simulink library "cube_lib"  (R2016a)
settings: Solver=VariableStepAuto  StartTime=0.0  StopTime=10.0  RelTol=1e-3
undefined symbols (not defined in the file): noise_standard_deviation, T_test_sensor, test_sensor_seed
libraries: simulink x2
settings Model: Creator=Stefan  LastModifiedBy=Love
settings DataIOCC: LimitDataPoints=on
settings DebuggingCC: AllowSymbolicDim=off
settings ModelReferenceCC: PropagateSignalLabelsOutOfModel=off
settings GRTTargetCC: GeneratePreprocessorConditionals=Use local settings

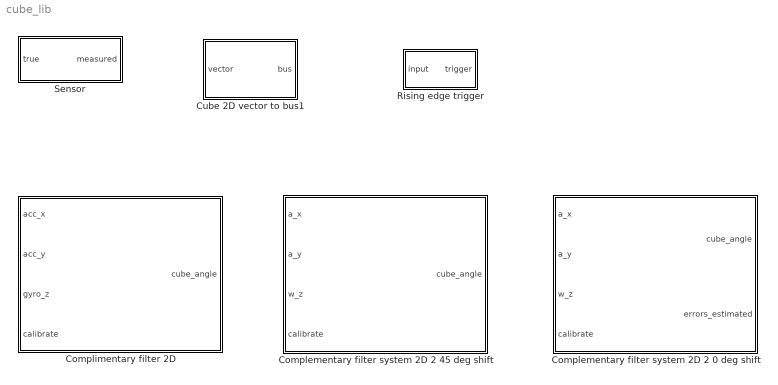
== system cube_lib ==
  Complementary filter system 2D 2 0 deg shift : Subsystem
  Complementary filter system 2D 2 45 deg shift : Subsystem
  Complimentary filter 2D : Subsystem
  Cube 2D vector to bus1 : Subsystem
  Rising edge trigger : Subsystem
  Sensor : Subsystem  mask{scale_factor=1, bias=0, noise_std=noise_standard_deviation, noise_seed=test_sensor_seed, sample_time=T_test_sensor}
      mask prompts: scale_factor "Scale factor"; noise_std "Noise standard deviation"; noise_seed "Noise seed"; sample_time "Sample time"
      mask help:
      | Simulates measurement by adding scale factor error, bias error and noise. Default sensor is a perfect sensor with sampling frequency 10 Hz.
      | Scale factor: 1
      | Bias: 0
      | Noise standard deviation: 0
      |
      | The sensor block contains the "Band-Limited White Noise" block which uses noise power instead of noise standard deviation. Noise power has the following definition:
      | noise_power = T_sample*standard_deviation^2
      | The white noise block has a correlation time of 0, meaning that all values are independent of each other, that is, white noise. (Simulink documentation for this block is confusion on this topic.)
      |
      | Due to the noise generator, sample time cannot be inherited.
      mask Callback sample_time:
      | sample_time_local = str2num(get_param(gcb,'sample_time'));
      | 
      | if sample_time_local <= 0
      |     msgbox(['Invalid setting for sample_time' char(10) ...
      |         'Due to noise generator, sample time cannot be inherited' char(10)...
      |         '(Yes, I know, it''s stupid!)']...
      |         ,'Error','error');
      |     set_param(gcb,'sample_time',num2str(0.1));
      | end

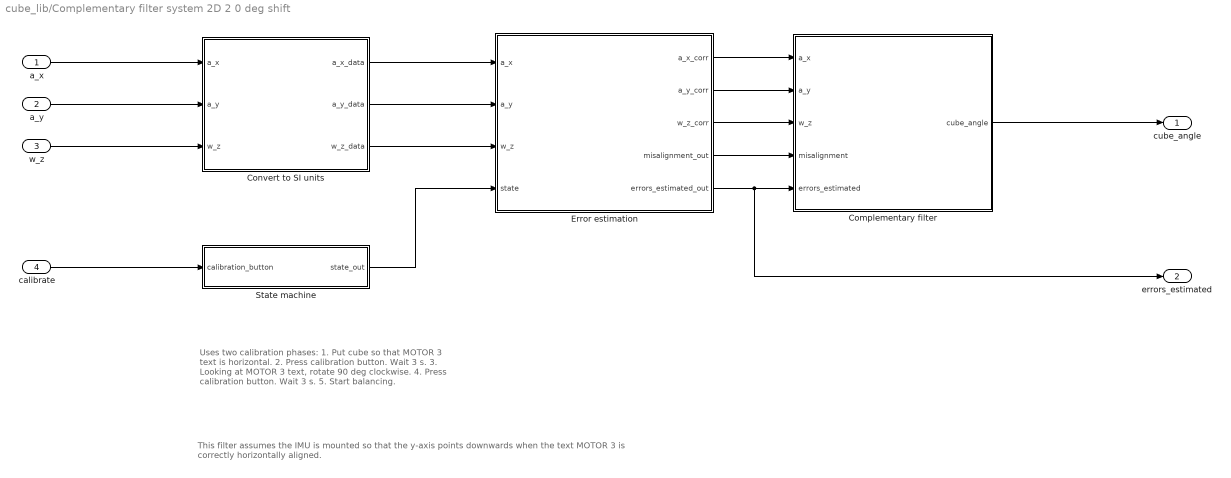
== system cube_lib/Complementary filter system 2D 2 0 deg shift ==
  note: This filter assumes the IMU is mounted so that the y-axis points downwards when the text MOTOR 3 is correctly horizontally aligned.
  note: Uses two calibration phases:
      | 1. Put cube so that MOTOR 3 text is horizontal.
      | 2. Press calibration button. Wait 3 s.
      | 3. Looking at MOTOR 3 text, rotate 90 deg clockwise.
      | 4. Press calibration button. Wait 3 s.
      | 5. Start balancing.
  a_x : Inport
  a_y : Inport  Port=2
  w_z : Inport  Port=3
  calibrate : Inport  Port=4
  Complementary filter : MATLAB Function  TreatAsAtomicUnit=on
  Convert to SI units : MATLAB Function  TreatAsAtomicUnit=on
  Error estimation : MATLAB Function  TreatAsAtomicUnit=on
  State machine : MATLAB Function  TreatAsAtomicUnit=on
  cube_angle : Outport
  errors_estimated : Outport  Port=2
  wires:
  Complementary filter/1(cube_angle) -> cube_angle/1
  w_z/1 -> Convert to SI units/3(w_z)
  a_x/1 -> Convert to SI units/1(a_x)
  a_y/1 -> Convert to SI units/2(a_y)
  Convert to SI units/1(a_x_data) -> Error estimation/1(a_x)
  Convert to SI units/2(a_y_data) -> Error estimation/2(a_y)
  Convert to SI units/3(w_z_data) -> Error estimation/3(w_z)
  Error estimation/1(a_x_corr) -> Complementary filter/1(a_x)
  Error estimation/5(errors_estimated_out) -> Complementary filter/5(errors_estimated), errors_estimated/1
  Error estimation/2(a_y_corr) -> Complementary filter/2(a_y)
  Error estimation/3(w_z_corr) -> Complementary filter/3(w_z)
  Error estimation/4(misalignment_out) -> Complementary filter/4(misalignment)
  calibrate/1 -> State machine/1(calibration_button)
  State machine/1(state_out) -> Error estimation/4(state)

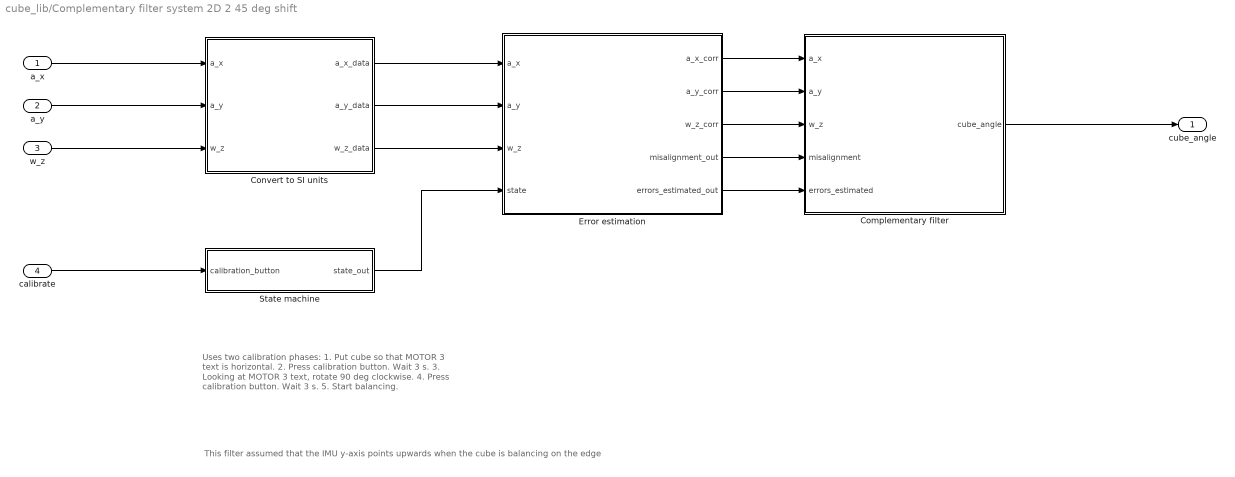
== system cube_lib/Complementary filter system 2D 2 45 deg shift ==
  note: This filter assumed that the IMU y-axis points upwards when the cube is balancing on the edge
  note: Uses two calibration phases:
      | 1. Put cube so that MOTOR 3 text is horizontal.
      | 2. Press calibration button. Wait 3 s.
      | 3. Looking at MOTOR 3 text, rotate 90 deg clockwise.
      | 4. Press calibration button. Wait 3 s.
      | 5. Start balancing.
  a_x : Inport
  a_y : Inport  Port=2
  w_z : Inport  Port=3
  calibrate : Inport  Port=4
  Complementary filter : MATLAB Function  TreatAsAtomicUnit=on
  Convert to SI units : MATLAB Function  TreatAsAtomicUnit=on
  Error estimation : MATLAB Function  TreatAsAtomicUnit=on
  State machine : MATLAB Function  TreatAsAtomicUnit=on
  cube_angle : Outport
  wires:
  State machine/1(state_out) -> Error estimation/4(state)
  calibrate/1 -> State machine/1(calibration_button)
  Error estimation/4(misalignment_out) -> Complementary filter/4(misalignment)
  Error estimation/3(w_z_corr) -> Complementary filter/3(w_z)
  Error estimation/2(a_y_corr) -> Complementary filter/2(a_y)
  Complementary filter/1(cube_angle) -> cube_angle/1
  Error estimation/5(errors_estimated_out) -> Complementary filter/5(errors_estimated)
  Error estimation/1(a_x_corr) -> Complementary filter/1(a_x)
  Convert to SI units/3(w_z_data) -> Error estimation/3(w_z)
  Convert to SI units/2(a_y_data) -> Error estimation/2(a_y)
  Convert to SI units/1(a_x_data) -> Error estimation/1(a_x)
  a_y/1 -> Convert to SI units/2(a_y)
  a_x/1 -> Convert to SI units/1(a_x)
  w_z/1 -> Convert to SI units/3(w_z)

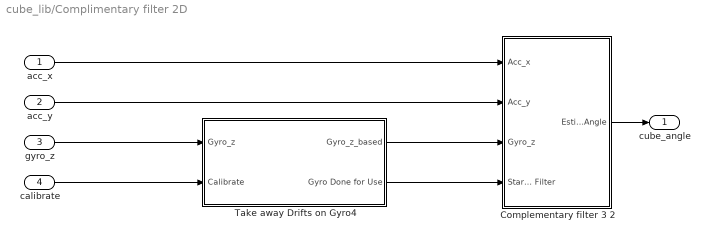
== system cube_lib/Complimentary filter 2D ==
  acc_x : Inport
  acc_y : Inport  Port=2
  gyro_z : Inport  Port=3
  calibrate : Inport  Port=4
  Complementary filter 3 2 : Subsystem
  Take away Drifts on Gyro4 : Subsystem
  cube_angle : Outport
  wires:
  calibrate/1 -> Take away Drifts on Gyro4/2(Calibrate)
  acc_y/1 -> Complementary filter 3 2/2(Acc_y)
  gyro_z/1 -> Take away Drifts on Gyro4/1(Gyro_z)
  acc_x/1 -> Complementary filter 3 2/1(Acc_x)
  Take away Drifts on Gyro4/2(Gyro Done for Use) -> Complementary filter 3 2/4("Start Complementary Filter ")
  Complementary filter 3 2/1(Estimated_Angle) -> cube_angle/1
  Take away Drifts on Gyro4/1(Gyro_z_based) -> Complementary filter 3 2/3(Gyro_z)

== system cube_lib/Cube 2D vector to bus1 ==
  vector : Inport
  Bus Creator1 : BusCreator  Inputs=5  OutDataTypeStr=Bus: CubeStates2D
  Demux2 : Demux  Outputs=5
  bus : Outport
  wires:
  vector/1 -> Demux2/1
  Demux2/3 -> Bus Creator1/3  "cube_angular_acceleration"
  Demux2/4 -> Bus Creator1/4  "wheel_angular_velocity"
  Demux2/5 -> Bus Creator1/5  "wheel_angular_acceleration"
  Demux2/2 -> Bus Creator1/2  "cube_angular_velocity"
  Demux2/1 -> Bus Creator1/1  "cube_angle"
  Bus Creator1/1 -> bus/1

== system cube_lib/Rising edge trigger ==
  input : Inport
  Compare To Zero : simulink/Logic and Bit Operations/Compare To Zero  relop=>  OutDataTypeStr=boolean
  Delay3 : Delay  DelayLength=1  InitialCondition=0
  Sum : Sum  Inputs=+-
  trigger : Outport
  wires:
  input/1 -> Sum/1, Delay3/1
  Delay3/1 -> Sum/2
  Compare To Zero/1 -> trigger/1
  Sum/1 -> Compare To Zero/1

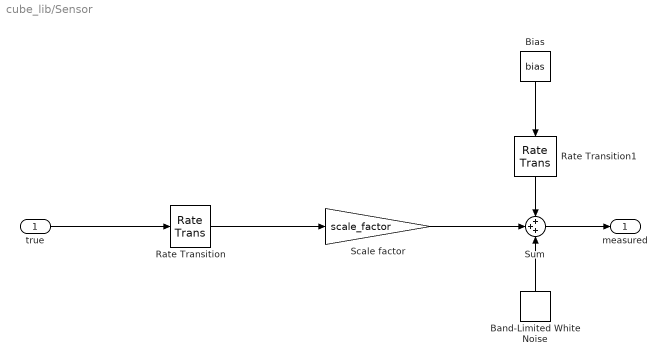
== system cube_lib/Sensor ==
  true : Inport
  Band-Limited White Noise : simulink/Sources/Band-Limited White Noise  Cov=sample_time*noise_std^2  Ts=sample_time  seed=noise_seed
  Bias : Constant  Value=bias
  Rate Transition : RateTransition  OutPortSampleTime=sample_time
  Rate Transition1 : RateTransition  OutPortSampleTime=sample_time
  Scale factor : Gain  Gain=scale_factor
  Sum : Sum  Inputs=+++
  measured : Outport
  wires:
  Rate Transition/1 -> Scale factor/1
  true/1 -> Rate Transition/1
  Sum/1 -> measured/1
  Scale factor/1 -> Sum/2
  Band-Limited White Noise/1 -> Sum/3
  Bias/1 -> Rate Transition1/1
  Rate Transition1/1 -> Sum/1

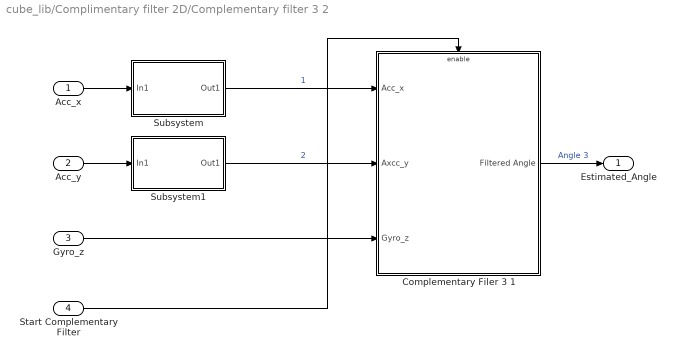
== system cube_lib/Complimentary filter 2D/Complementary filter 3 2 ==
  Acc_x : Inport
  Acc_y : Inport  Port=2
  Gyro_z : Inport  Port=3
  "Start Complementary Filter " : Inport  Port=4
  Complementary Filer 3 1 : Subsystem
  Subsystem : Subsystem
  Subsystem1 : Subsystem
  Estimated_Angle : Outport
  wires:
  Acc_x/1 -> Subsystem/1(In1)
  Acc_y/1 -> Subsystem1/1(In1)
  Complementary Filer 3 1/1(Filtered Angle) -> Estimated_Angle/1  "Angle 3"
  "Start Complementary Filter "/1 -> Complementary Filer 3 1/Enable
  Gyro_z/1 -> Complementary Filer 3 1/3(Gyro_z)
  Subsystem1/1(Out1) -> Complementary Filer 3 1/2(Axcc_y)  "2"
  Subsystem/1(Out1) -> Complementary Filer 3 1/1(Acc_x)  "1"

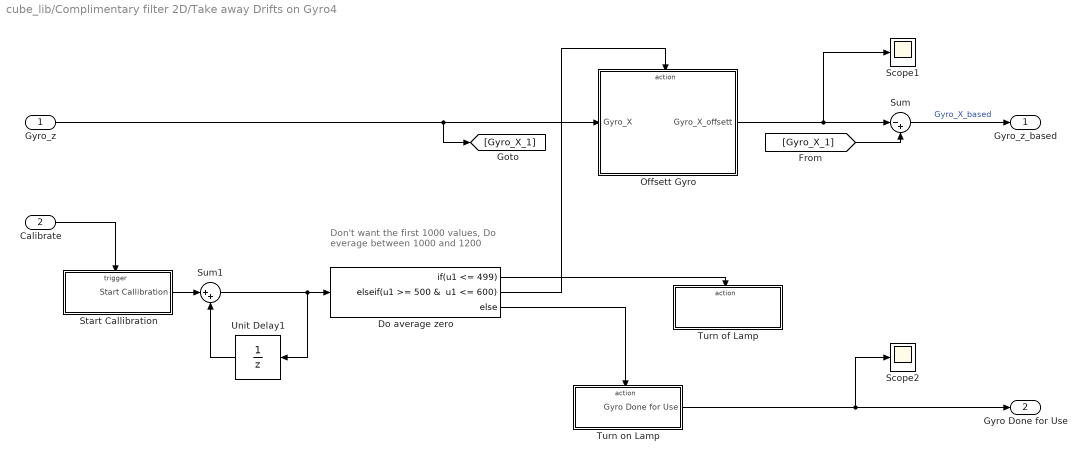
== system cube_lib/Complimentary filter 2D/Take away Drifts on Gyro4 ==
  note: Don't want the first 1000 values,
      | Do everage between 1000 and 1200
  Gyro_z : Inport
  Calibrate : Inport  Port=2
  Do average zero : If  IfExpression=u1 <= 499  ElseIfExpressions="u1 >= 500 &  u1 <= 600"
  Offsett Gyro : Subsystem
  Scope1 : Scope
  Scope2 : Scope
  Start Callibration : Subsystem
  Sum : Sum  Inputs=|-+
  Sum1 : Sum  Inputs=|++
  Turn of Lamp : Subsystem
  Turn on Lamp : Subsystem
  Unit Delay1 : UnitDelay  SampleTime=-1
  Gyro_z_based : Outport
  Gyro Done for Use : Outport  Port=2
  wires:
  Turn on Lamp/1(Gyro Done for Use) -> Gyro Done for Use/1, Scope2/1
  Do average zero/1 -> Turn of Lamp/Action
  Start Callibration/1(Start Callibration) -> Sum1/1
  Calibrate/1 -> Start Callibration/Trigger
  Do average zero/3 -> Turn on Lamp/Action
  Do average zero/2 -> Offsett Gyro/Action
  Gyro_z/1 -> Offsett Gyro/1(Gyro_X), [Gyro_X_1]
  Sum/1 -> Gyro_z_based/1  "Gyro_X_based"
  Offsett Gyro/1(Gyro_X_offsett) -> Sum/1, Scope1/1
  [Gyro_X_1] -> Sum/2
  Sum1/1 -> Unit Delay1/1, Do average zero/1
  Unit Delay1/1 -> Sum1/2

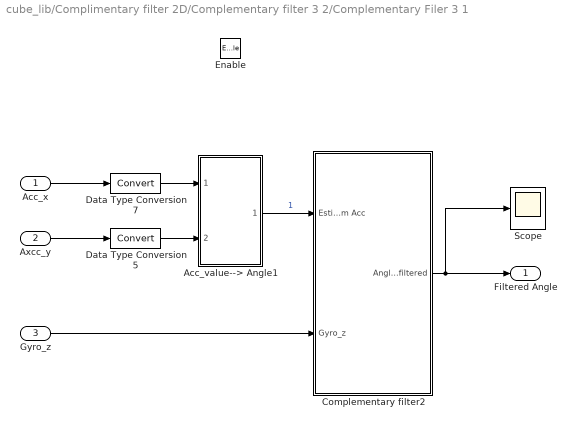
== system cube_lib/Complimentary filter 2D/Complementary filter 3 2/Complementary Filer 3 1 ==
  Acc_x : Inport
  Axcc_y : Inport  Port=2
  Gyro_z : Inport  Port=3
  Enable : EnablePort  StatesWhenEnabling=reset
  Acc_value--> Angle1 : Subsystem
  Complementary filter2 : Subsystem
  Data Type Conversion5 : DataTypeConversion
  Data Type Conversion7 : DataTypeConversion
  Scope : Scope
  Filtered Angle : Outport  OutputWhenDisabled=reset  InitialOutput=[0]
  wires:
  Gyro_z/1 -> Complementary filter2/2(Gyro_z)
  Data Type Conversion5/1 -> Acc_value--> Angle1/2(Acc_y)
  Data Type Conversion7/1 -> Acc_value--> Angle1/1(Acc_x)
  Axcc_y/1 -> Data Type Conversion5/1
  Acc_value--> Angle1/1(Angle) -> Complementary filter2/1(Estimated angle from Acc)  "1"
  Acc_x/1 -> Data Type Conversion7/1
  Complementary filter2/1(Angle_filtered) -> Filtered Angle/1, Scope/1

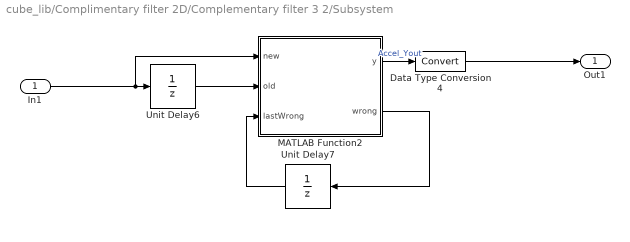
== system cube_lib/Complimentary filter 2D/Complementary filter 3 2/Subsystem ==
  In1 : Inport
  Data Type Conversion4 : DataTypeConversion
  MATLAB Function2 : MATLAB Function  TreatAsAtomicUnit=on
  Unit Delay6 : UnitDelay  InitialCondition=-40.45  SampleTime=-1
  Unit Delay7 : UnitDelay  SampleTime=-1
  Out1 : Outport
  wires:
  In1/1 -> Unit Delay6/1, MATLAB Function2/1(new)
  MATLAB Function2/1(y) -> Data Type Conversion4/1  "Accel_Yout"
  MATLAB Function2/2(wrong) -> Unit Delay7/1
  Unit Delay6/1 -> MATLAB Function2/2(old)
  Unit Delay7/1 -> MATLAB Function2/3(lastWrong)
  Data Type Conversion4/1 -> Out1/1

== system cube_lib/Complimentary filter 2D/Complementary filter 3 2/Subsystem1 ==
  In1 : Inport
  Data Type Conversion4 : DataTypeConversion
  MATLAB Function2 : MATLAB Function  TreatAsAtomicUnit=on
  Unit Delay6 : UnitDelay  InitialCondition=-40.45  SampleTime=-1
  Unit Delay7 : UnitDelay  SampleTime=-1
  Out1 : Outport
  wires:
  In1/1 -> Unit Delay6/1, MATLAB Function2/1(new)
  MATLAB Function2/1(y) -> Data Type Conversion4/1  "Accel_Yout"
  MATLAB Function2/2(wrong) -> Unit Delay7/1
  Unit Delay6/1 -> MATLAB Function2/2(old)
  Unit Delay7/1 -> MATLAB Function2/3(lastWrong)
  Data Type Conversion4/1 -> Out1/1

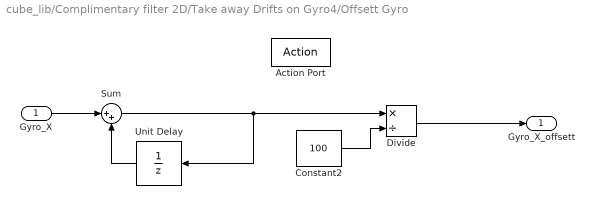
== system cube_lib/Complimentary filter 2D/Take away Drifts on Gyro4/Offsett Gyro ==
  Gyro_X : Inport
  Action Port : ActionPort
  Constant2 : Constant  Value=100
  Divide : Product  Inputs=*/
  Sum : Sum  Inputs=|++
  Unit Delay : UnitDelay  SampleTime=-1
  Gyro_X_offsett : Outport
  wires:
  Sum/1 -> Unit Delay/1, Divide/1
  Divide/1 -> Gyro_X_offsett/1
  Gyro_X/1 -> Sum/1
  Constant2/1 -> Divide/2
  Unit Delay/1 -> Sum/2

== system cube_lib/Complimentary filter 2D/Take away Drifts on Gyro4/Start Callibration ==
  Trigger : TriggerPort  VariantControl=Variant  PortDimensions=1
  Constant2 : Constant
  Start Callibration : Outport  InitialOutput=[0]
  wires:
  Constant2/1 -> Start Callibration/1

== system cube_lib/Complimentary filter 2D/Take away Drifts on Gyro4/Turn of Lamp ==
  Action Port : ActionPort

== system cube_lib/Complimentary filter 2D/Take away Drifts on Gyro4/Turn on Lamp ==
  Action Port : ActionPort
  Constant6 : Constant  SampleTime=-1
  Gyro Done for Use : Outport  InitialOutput=[0]
  wires:
  Constant6/1 -> Gyro Done for Use/1

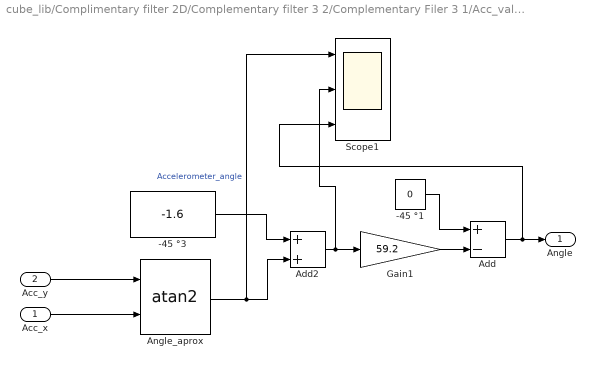
== system cube_lib/Complimentary filter 2D/Complementary filter 3 2/Complementary Filer 3 1/Acc_value--> Angle1 ==
  Acc_x : Inport
  Acc_y : Inport  Port=2
  -45 °1 : Constant  Value=0
  -45 °3 : Constant  Value=-1.6
  Add : Sum  Inputs=+-
  Add2 : Sum
  Angle_aprox : Trigonometry  Operator=atan2
  Gain1 : Gain  Gain=59.2
  Scope1 : Scope  NumInputPorts=3
  Angle : Outport
  wires:
  Add2/1 -> Gain1/1, Scope1/2
  Angle_aprox/1 -> Add2/2, Scope1/1  "Accelerometer_angle"
  -45 °3/1 -> Add2/1
  -45 °1/1 -> Add/1
  Add/1 -> Angle/1, Scope1/3
  Gain1/1 -> Add/2
  Acc_x/1 -> Angle_aprox/2
  Acc_y/1 -> Angle_aprox/1

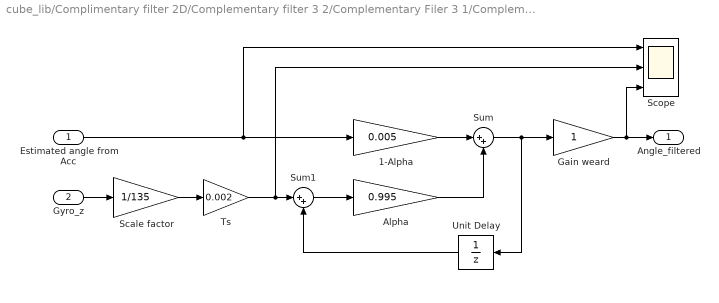
== system cube_lib/Complimentary filter 2D/Complementary filter 3 2/Complementary Filer 3 1/Complementary filter2 ==
  Estimated angle from Acc : Inport
  Gyro_z : Inport  Port=2
  1-Alpha : Gain  Gain=0.005
  Alpha : Gain  Gain=0.995
  Gain weard : Gain
  Scale factor : Gain  Gain=1/135
  Scope : Scope  NumInputPorts=3
  Sum : Sum  Inputs=|++
  Sum1 : Sum  Inputs=|++
  Ts : Gain  Gain=0.002
  Unit Delay : UnitDelay  SampleTime=-1
  Angle_filtered : Outport
  wires:
  Scale factor/1 -> Ts/1
  Sum/1 -> Unit Delay/1, Gain weard/1
  Gain weard/1 -> Scope/3, Angle_filtered/1
  Estimated angle from Acc/1 -> 1-Alpha/1, Scope/1
  Gyro_z/1 -> Scale factor/1
  Unit Delay/1 -> Sum1/2
  Alpha/1 -> Sum/2
  Sum1/1 -> Alpha/1
  Ts/1 -> Sum1/1, Scope/2
  1-Alpha/1 -> Sum/1

== matlab function cube_lib/Complementary filter system 2D 2 0 deg shift/Complementary filter ==
  data: a_x input size=1; a_y input size=1; w_z input size=1; misalignment input size=1; cube_angle output; errors_estimated input size=1
function cube_angle = ComplementaryFilter(a_x,a_y,w_z,misalignment,errors_estimated)
%#codegen
% Uses the equation:
% theta(k) = alfa*(theta(k-1) + w_z*T) + (1-alfa)*a(k);
% where a(k) is the estimated angle from the accelerometers
%
% alfa from cubeparameters

persistent theta_k_1; % Previous cube angle
persistent initiate_filter;

alfa = 0.995;
T_onboard = 0.002;
angle_correction = 135*pi/180; % Due to mounting

if isempty(theta_k_1)
    initiate_filter = 1;
    theta_k_1 = 0;
end

if errors_estimated && initiate_filter % First call to complementary filter (when no previous value exists)
    theta = atan2(a_x,a_y)-misalignment;
    initiate_filter = 0;
elseif errors_estimated
    % Complementary filter
    a_k = atan2(a_x,a_y)-misalignment; % Angle estimation from accelerometers
    % Improvement: Compensate for angular acceleration and centripetal
    % force
    theta = alfa*(theta_k_1 + w_z*T_onboard) + (1-alfa)*a_k;
else
    theta = 0;
end

theta_k_1 = theta;  % Save value

% Assign output
if errors_estimated
    cube_angle = theta + angle_correction;
else
    cube_angle = 0;
end

== matlab function cube_lib/Complementary filter system 2D 2 0 deg shift/Convert to SI units ==
  data: a_x input; a_x_data output double; a_y input; w_z input; a_y_data output double; w_z_data output double
function [a_x_data,a_y_data,w_z_data] = ConvertImuData(a_x,a_y,w_z)
%#codegen

g_ = 9.81*m_/s_^2;
a_scale_factor = 16384; % AFS_SEL = 0, se datablad MPU9250
w_scale_factor = 131;   % FS_SEL = 0, se datablad MPU9250
a_x_data = double(a_x)/a_scale_factor*g_;
a_y_data = double(a_y)/a_scale_factor*g_;
w_z_data = double(w_z)/w_scale_factor*deg_;

== matlab function cube_lib/Complementary filter system 2D 2 0 deg shift/Error estimation ==
  data: a_x input; a_x_corr output; a_y_corr output; w_z_corr output; misalignment_out output; a_y input; w_z input; state input; errors_estimated_out output
function [a_x_corr,a_y_corr,w_z_corr,misalignment_out,errors_estimated_out] = ErrorEstimatedImu(a_x,a_y,w_z,state)
%#codegen
% Finds IMU errors and corrects IMU data
persistent a_x_1; % Vector
persistent a_x_2; % Vector
persistent a_y_1; % Vector
persistent a_y_2; % Vector
persistent w_z_1; % Vector
persistent w_z_2; % Vector
persistent w_z_turn; % Scalar (sum)
persistent n_samples_w_z_turn; % Counts number of samples used for turn to compensate for bias
persistent k_sample;
persistent previous_state;
persistent errors_estimated;
persistent bias_a_x;
persistent bias_a_y;
persistent bias_w_z;
persistent scale_factor_a_x;
persistent scale_factor_a_y;
persistent scale_factor_w_z;
persistent misalignment;

n_samples = 1000; % Two seconds with T=0.002. Hardcoded for compiler
T_onboard = 0.002; % So that it does not have to be input or a set parameter

if isempty(a_x_1)
    k_sample = 1;
    previous_state = 0;
    errors_estimated = 0;
    a_x_1 = zeros(n_samples,1);
    a_x_2 = zeros(n_samples,1);
    a_y_1 = zeros(n_samples,1);
    a_y_2 = zeros(n_samples,1);
    w_z_1 = zeros(n_samples,1);
    w_z_2 = zeros(n_samples,1);
    w_z_turn = 0;
    n_samples_w_z_turn = 0;
    bias_a_x = 0;
    bias_a_y = 0;
    bias_w_z = 0;
    scale_factor_a_x = 0;
    scale_factor_a_y = 0;
    scale_factor_w_z = 0;
    misalignment = 0;
end

if state ~= previous_state % Entering a new state
    k_sample = 1;
    if state == 0 % Start over
        errors_estimated = 0;
        a_x_1 = zeros(n_samples,1);
        a_x_2 = zeros(n_samples,1);
        a_y_1 = zeros(n_samples,1);
        a_y_2 = zeros(n_samples,1);
        w_z_1 = zeros(n_samples,1);
        w_z_2 = zeros(n_samples,1);
        w_z_turn = 0;
        n_samples_w_z_turn = 0;
        bias_a_x = 0;
        bias_a_y = 0;
        bias_w_z = 0;
        scale_factor_a_x = 0;
        scale_factor_a_y = 0;
        scale_factor_w_z = 0;
        misalignment = 0;
    end
end

% Collect data in two phases, where cube_angle = -45 deg and cube_angle = 45 deg
if state == 1 && k_sample <= n_samples
    a_x_1(k_sample) = a_x;
    a_y_1(k_sample) = a_y;
    w_z_1(k_sample) = w_z;
    k_sample = k_sample + 1;
elseif state == 1
    w_z_turn = w_z_turn + w_z;
    n_samples_w_z_turn = n_samples_w_z_turn + 1;
    
end

if state == 2 && k_sample <= n_samples
    a_x_2(k_sample) = a_x;
    a_y_2(k_sample) = a_y;
    w_z_2(k_sample) = w_z;
    k_sample = k_sample + 1;
end

% Estimate errors when data from the two fixed positions have been done
if state == 2 && k_sample > n_samples && ~errors_estimated % We can estimate the errors
    % Sections
    a_x_1_meas = mean(a_x_1);
    a_x_2_meas = mean(a_x_2);
    a_y_1_meas = mean(a_y_1);
    a_y_2_meas = mean(a_y_2);
    w_z_meas   = mean([w_z_1;w_z_2]);
    
    % Call error estimation function
    % Derive expressions from this equations system:
    %  / a_1_measured = scale_factor*a_2_true + bias
    % {
    %  \ a_2_measured = scale_factor*a_2_true + bias
    g = 9.81;
    
    % IMU aligned with cube side, so that the y-axis points downwards when
    % the text MOTOR 3 is correctly horizontally aligned
    % First position:  a_x = 0, a_y = g
    % Second position: a_x = g, a_y = 0
    % That means:
    % a_x_1_meas = bias_x
    % a_x_2_meas = scale_factor_x*-g+bias_x = scale_factor_x*-g + a_x_1_meas
    %   and
    % a_y_1_meas = scale_factor_y*-g+bias_y = scale_factor_y*-g + a_y_1_meas
    % a_y_2_meas = bias_y
    % Great!
    bias_a_x = a_x_1_meas;
    bias_a_y = a_y_2_meas;
    scale_factor_a_x = (a_x_1_meas-a_x_2_meas)/g;
    scale_factor_a_y = (a_y_2_meas-a_y_1_meas)/g;
    
    % Gyro
    bias_w_z = w_z_meas; % Cube is still. What is measured is bias (and error)
    scale_factor_w_z = w_z_turn*T_onboard/(pi/2)-n_samples_w_z_turn*bias_w_z*T_onboard/(pi/2); % Should be a pi/2 turn. Compensate for bias.
    
    % Misalignment
    misalignment = 0;
    
    errors_estimated = 1;
end

% Update
previous_state = state;

% Assign output
if errors_estimated
    a_x_corr = (a_x-bias_a_x)/scale_factor_a_x;
    a_y_corr = (a_y-bias_a_y)/scale_factor_a_y;
    w_z_corr = (w_z-bias_w_z)/scale_factor_w_z;
else
    a_x_corr = a_x;
    a_y_corr = a_y;
    w_z_corr = w_z;
end

misalignment_out = misalignment;
errors_estimated_out = errors_estimated;

== matlab function cube_lib/Complementary filter system 2D 2 0 deg shift/State machine ==
  data: calibration_button input; state_out output
function state_out = StateMachine(calibration_button)
%#codegen
% Step between states 0, 1 and 2 from calibration button

persistent previous_value;
persistent sample;
persistent state;
persistent button_released;

min_samples_between_state_shift = 500; % 500 = 1 s

if isempty(previous_value)
    previous_value = false;
    state = 0;
    sample = min_samples_between_state_shift; % So that button can be clicked instantly
    button_released = true; % Button should be released inbetween clicks
end

if previous_value == 0 && calibration_button == 1 && sample > min_samples_between_state_shift && button_released
    state = state + 1;
    sample = 0;
    button_released = false;
end

if state == 3 % Start over
    state = 0;
end

if previous_value == 1 && calibration_button == 0
    button_released = true;
end

% Increment
sample = sample + 1;
previous_value = calibration_button;

% Assign output
state_out = state;

== matlab function cube_lib/Complementary filter system 2D 2 45 deg shift/Complementary filter ==
  data: a_x input size=1; a_y input size=1; w_z input size=1; misalignment input size=1; cube_angle output; errors_estimated input size=1
function cube_angle = ComplementaryFilter(a_x,a_y,w_z,misalignment,errors_estimated)
%#codegen
% Uses the equation:
% theta(k) = alfa*(theta(k-1) + w_z*T) + (1-alfa)*a(k);
% where a(k) is the estimated angle from the accelerometers
%
% alfa from cubeparameters

persistent theta_k_1; % Previous cube angle
persistent initiate_filter;

alfa = 0.995;
T_onboard = 0.002;

if isempty(theta_k_1)
    initiate_filter = 1;
    theta_k_1 = 0;
end

if errors_estimated && initiate_filter % First call to complementary filter (when no previous value exists)
    theta = atan2(a_x,a_y)-misalignment;
    initiate_filter = 0;
elseif errors_estimated
    % Complementary filter
    a_k = atan2(a_x,a_y)-misalignment; % Angle estimation from accelerometers
    % Improvement: Compensate for angular acceleration and centripetal
    % force
    theta = alfa*(theta_k_1 + w_z*T_onboard) + (1-alfa)*a_k;
else
    theta = 0;
end

theta_k_1 = theta;  % Save value

% Assign output
cube_angle = theta;

== matlab function cube_lib/Complementary filter system 2D 2 45 deg shift/Convert to SI units ==
  data: a_x input; a_x_data output double; a_y input; w_z input; a_y_data output double; w_z_data output double
function [a_x_data,a_y_data,w_z_data] = ConvertImuData(a_x,a_y,w_z)
%#codegen

g_ = 9.81*m_/s_^2;
a_scale_factor = 16384; % AFS_SEL = 0, se datablad MPU9250
w_scale_factor = 131;   % FS_SEL = 0, se datablad MPU9250
a_x_data = double(a_x)/a_scale_factor*g_;
a_y_data = double(a_y)/a_scale_factor*g_;
w_z_data = double(w_z)/w_scale_factor*deg_;

== matlab function cube_lib/Complementary filter system 2D 2 45 deg shift/Error estimation ==
  data: a_x input; a_x_corr output; a_y_corr output; w_z_corr output; misalignment_out output; a_y input; w_z input; state input; errors_estimated_out output
function [a_x_corr,a_y_corr,w_z_corr,misalignment_out,errors_estimated_out] = ErrorEstimatedImu(a_x,a_y,w_z,state)
%#codegen
% Finds IMU errors and corrects IMU data
persistent a_x_1;
persistent a_x_2;
persistent a_y_1;
persistent a_y_2;
persistent w_z_1;
persistent w_z_2;
persistent k_sample;
persistent previous_state;
persistent errors_estimated;
persistent bias_a_x;
persistent bias_a_y;
persistent bias_w_z;
persistent scale_factor_a_x;
persistent scale_factor_a_y;
persistent scale_factor_w_z;
persistent misalignment;

n_samples = 1000; % Two seconds with T=0.002. Hardcoded for compiler

if isempty(a_x_1)
    k_sample = 1;
    previous_state = 0;
    errors_estimated = 0;
    a_x_1 = zeros(n_samples,1);
    a_x_2 = zeros(n_samples,1);
    a_y_1 = zeros(n_samples,1);
    a_y_2 = zeros(n_samples,1);
    w_z_1 = zeros(n_samples,1);
    w_z_2 = zeros(n_samples,1);
    bias_a_x = 0;
    bias_a_y = 0;
    bias_w_z = 0;
    scale_factor_a_x = 0;
    scale_factor_a_y = 0;
    scale_factor_w_z = 0;
    misalignment = 0;
end

if state ~= previous_state % Entering a new state
    k_sample = 1;
end

% Collect data in two sections, where cube_angle = 45 deg and cube_angle = -45 deg
if state == 1 && k_sample <= n_samples
    a_x_1(k_sample) = a_x;
    a_y_1(k_sample) = a_y;
    w_z_1(k_sample) = w_z;
    k_sample = k_sample + 1;
end

if state == 2 && k_sample <= n_samples
    a_x_2(k_sample) = a_x;
    a_y_2(k_sample) = a_y;
    w_z_2(k_sample) = w_z;
    k_sample = k_sample + 1;
end

% Estimate errors when data from the two fixed positions have been done
if state == 2 && k_sample > n_samples && ~errors_estimated % We can estimate the errors
    % Sections
    a_x_1_meas = mean(a_x_1);
    a_x_2_meas = mean(a_x_2);
    a_y_1_meas = mean(a_y_1);
    a_y_2_meas = mean(a_y_2);
    w_z_meas   = mean([w_z_1;w_z_2]);
    
    % Call error estimation function
    [misalignment,...
     bias_a_x,...
     bias_a_y,...
     bias_w_z,...
     scale_factor_a_x,...
     scale_factor_a_y,...
     scale_factor_w_z] = CalculateImuErrors2D(a_x_1_meas,...
                                              a_x_2_meas,...
                                              a_y_1_meas,...
                                              a_y_2_meas,...
                                              w_z_meas);

    errors_estimated = 1;
end

% Update
previous_state = state;

% Assign output
if errors_estimated
    a_x_corr = (a_x-bias_a_x)/scale_factor_a_x;
    a_y_corr = (a_y-bias_a_y)/scale_factor_a_y;
    w_z_corr = (w_z-bias_w_z)/scale_factor_w_z;
else
    a_x_corr = a_x;
    a_y_corr = a_y;
    w_z_corr = w_z;
end

misalignment_out = misalignment;
errors_estimated_out = errors_estimated;

== matlab function cube_lib/Complementary filter system 2D 2 45 deg shift/State machine ==
  data: calibration_button input; state_out output
function state_out = StateMachine(calibration_button)
%#codegen

persistent previous_value;
persistent sample;
persistent state;
persistent button_released;

min_samples_between_state_shift = 500; % 500 = 1 s

if isempty(previous_value)
    previous_value = false;
    state = 0;
    sample = min_samples_between_state_shift; % So that button can be clicked instantly
    button_released = true; % Button should be released inbetween clicks
end

if previous_value == 0 && calibration_button == 1 && sample > min_samples_between_state_shift && button_released
    state = state + 1;
    sample = 0;
    button_released = false;
end

if previous_value == 1 && calibration_button == 0
    button_released = true;
end

% Increment
sample = sample + 1;
previous_value = calibration_button;

% Assign output
state_out = state;

== matlab function cube_lib/Complimentary filter 2D/Complementary filter 3 2/Subsystem/MATLAB Function2 ==
  data: y output; new input; old input; wrong output; lastWrong input
function [y, wrong]= fcn(new, old, lastWrong)
%#codegen
if(old-new > 4000 || new-old > 4000)
    if(lastWrong == 1)
        y = new;
        wrong = 0;
    else
        y = old;
        wrong = 1;
    end
else
    y = new;
    wrong = 0;
end

== matlab function cube_lib/Complimentary filter 2D/Complementary filter 3 2/Subsystem1/MATLAB Function2 ==
  data: y output; new input; old input; wrong output; lastWrong input
function [y, wrong]= fcn(new, old, lastWrong)
%#codegen
if(old-new > 4000 || new-old > 4000)
    if(lastWrong == 1)
        y = new;
        wrong = 0;
    else
        y = old;
        wrong = 1;
    end
else
    y = new;
    wrong = 0;
end
